simulink model "sl_subsys_fcncall5"  (Simulink 7.6)
settings: Solver=FixedStepDiscrete  StartTime=0.0  StopTime=10.0  FixedStep=1  RelTol=1e-3
Description:
  | Multiple initiators of a function-call subsystem
  | 
  | The following function-call subsystem is called by two different function-call
  | initiators (Chart1 and Chart2). The data connection between Chart1/out1 and
  | Chart2/d1 guarantees that Chart1 executes before Chart2.
  | 
  | Caution needs to be taken when creating function-call subsystems with
  | multiple callers. For example, if you remove the data connection between Chart1 and
  | Chart2, then you need to add priorities to Chart1 and Chart2 using the block
  | property dialogs to specify the relative execution order of these blocks. Failure
  | to do so will mean that your model's execution, in general, will be
  | ambiguous. However, Simulink does not error out for this condition because
  | it may be valid for specific cases. As an example, if all states are removed from
  | f() and the line from Chart1/out1 to Chart2/d1 is deleted, then the order in which
  | Chart1 and Chart2 execute does not matter.
settings Model: Creator=The MathWorks Inc.  CovMetricSettings=d  ExtModeAutoUpdateStatusClock=off
settings OptimizationCC: BlockReduction=off  BooleanDataType=off  InlineInvariantSignals=on  InitFltsAndDblsToZero=on
settings DebuggingCC: SaveWithParameterizedLinksMsg=none  SignalResolutionControl=TryResolveAllWithWarning  SolverPrmCheckMsg=none  MultiTaskDSMMsg=warning  MultiTaskCondExecSysMsg=none
settings HardwareCC: TargetUnknown=on
settings SFSimCC: SimParseCustomCode=off
settings RTWCC: IncludeERTFirstTime=on
settings CodeAppCC: CustomSymbolStrFcn=$F$N$M
settings GRTTargetCC: TargetFcnLib=ansi_tfl_tmw.mat

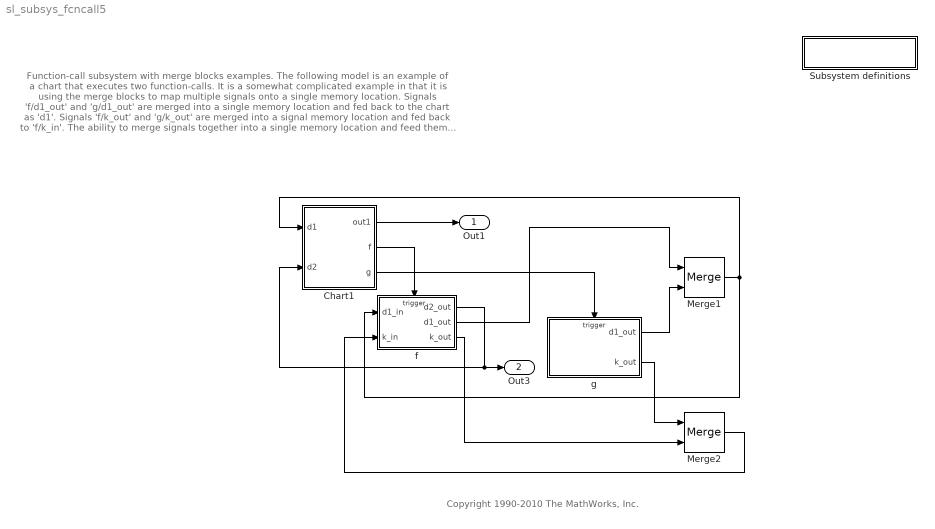
== system sl_subsys_fcncall5 ==
  note: Function-call subsystem with merge blocks examples.
      |
      | The following model is an example of a chart that executes two function-calls.
      | It is a somewhat complicated example in that it is using the merge blocks to
      | map multiple signals onto a single memory location. Signals 'f/d1_out' and
      | 'g/d1_out' are merged into a single memory location and fed back to the chart
      | as 'd1'. Signals 'f/k_out' and 'g/k_out' are merged into a signal memory
      | location and fed back to 'f/k_in'. The ability to merge signals together
      | into a single memory location and feed them back to the chart enables the
      | Chart to make complex decisions about how to compute values.
  note: Copyright 1990-2010 The MathWorks, Inc.
  " Subsystem definitions" : Subsystem
      settings: OpenFcn=helpview([matlabroot,'/toolbox/simulink/simdemos/simfeatures/html/sl_subsys_definitions.html']);
      mask Display: disp('Subsystem\ndefinitions')
  Chart1 : Stateflow chart  TreatAsAtomicUnit=on
  Merge1 : Merge
  Merge2 : Merge
  f : Subsystem  TreatAsAtomicUnit=on
  g : Subsystem  TreatAsAtomicUnit=on
  Out1 : Outport
  Out3 : Outport  Port=2
  wires:
  Chart1/2(f) -> f/Trigger
  f/1(d2_out) -> Out3/1, Chart1/2(d2)
  g/1(d1_out) -> Merge1/2
  Chart1/1(out1) -> Out1/1
  Chart1/3(g) -> g/Trigger
  f/2(d1_out) -> Merge1/1
  Merge1/1 -> f/1(d1_in), Chart1/1(d1)
  f/3(k_out) -> Merge2/2
  g/2(k_out) -> Merge2/1
  Merge2/1 -> f/2(k_in)

== system sl_subsys_fcncall5/ Subsystem definitions ==

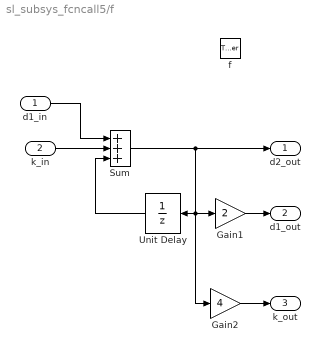
== system sl_subsys_fcncall5/f ==
  d1_in : Inport
  k_in : Inport  Port=2
  f : TriggerPort  TriggerType=function-call
  Gain1 : Gain  Gain=2  SaturateOnIntegerOverflow=on  OutDataTypeStr=Inherit: Same as input  ParamDataTypeStr=Inherit: Same as input
  Gain2 : Gain  Gain=4  SaturateOnIntegerOverflow=on  OutDataTypeStr=Inherit: Same as input  ParamDataTypeStr=Inherit: Same as input
  Sum : Sum  Inputs=+++  SaturateOnIntegerOverflow=on  InputSameDT=on  OutDataTypeStr=Inherit: Same as first input
  Unit Delay : UnitDelay  SampleTime=-1
  d2_out : Outport
  d1_out : Outport  Port=2
  k_out : Outport  Port=3
  wires:
  Unit Delay/1 -> Sum/3
  Sum/1 -> Unit Delay/1, Gain1/1, Gain2/1, d2_out/1
  d1_in/1 -> Sum/1
  Gain1/1 -> d1_out/1
  Gain2/1 -> k_out/1
  k_in/1 -> Sum/2

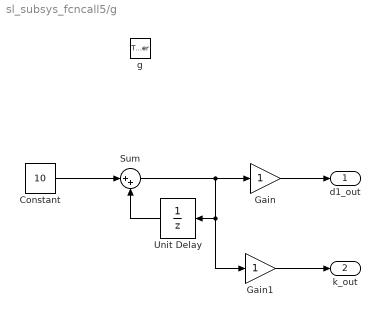
== system sl_subsys_fcncall5/g ==
  g : TriggerPort  TriggerType=function-call
  Constant : Constant  Value=10
  Gain : Gain  SaturateOnIntegerOverflow=on  OutDataTypeStr=Inherit: Same as input  ParamDataTypeStr=Inherit: Same as input
  Gain1 : Gain  SaturateOnIntegerOverflow=on  OutDataTypeStr=Inherit: Same as input  ParamDataTypeStr=Inherit: Same as input
  Sum : Sum  Inputs=|++  SaturateOnIntegerOverflow=on  InputSameDT=on  OutDataTypeStr=Inherit: Same as first input
  Unit Delay : UnitDelay  SampleTime=-1
  d1_out : Outport
  k_out : Outport  Port=2
  wires:
  Constant/1 -> Sum/1
  Unit Delay/1 -> Sum/2
  Sum/1 -> Gain/1, Unit Delay/1, Gain1/1
  Gain/1 -> d1_out/1
  Gain1/1 -> k_out/1

== stateflow chart Chart1 ==
  state one/
    entry: f; out1= d1+d2;
  state two/
    entry: g; out1=d1-d2;
  one -> two
  two -> one
  (default) -> one
  data: d1 input double; d2 input double; out1 output double
  events: f output FUNCTION_CALL_EVENT; g output FUNCTION_CALL_EVENT
